simulink model "MyComplexModel_V13R2023a"  (R2023a)
settings: Solver=ode23tb  StartTime=0.0  StopTime=30  FixedStep=0.001  MaxStep=0.001  RelTol=1e-6
values from neighbouring files (symbols this model uses):
  alpha_IS = 30 / (V30_IS.^beta_IS)    [run_one_case_conditional_sampling_pediatric_noVAD_linear.m]    (also in run_one_case_pediatric_noVAD_linear.m)
  alpha_LA = 30 / (V30_LA.^beta_LA)    [run_one_case_conditional_sampling_pediatric_noVAD_linear.m]    (also in run_one_case_pediatric_noVAD_linear.m)
  alpha_LV = 30 / (V30_LV.^beta_LV)    [run_one_case_conditional_sampling_pediatric_noVAD_linear.m]    (also in run_one_case_pediatric_noVAD_linear.m)
  alpha_RA = 30 / (V30_RA.^beta_RA)    [run_one_case_conditional_sampling_pediatric_noVAD_linear.m]    (also in run_one_case_pediatric_noVAD_linear.m)
  alpha_RV = 30 / (V30_RV.^beta_RV)    [run_one_case_conditional_sampling_pediatric_noVAD_linear.m]    (also in run_one_case_pediatric_noVAD_linear.m)
  beta_IS = (log(Pm_IS / 30)) / (log(Vm_IS / V30_IS))    [run_one_case_conditional_sampling_pediatric_noVAD_linear.m]    (also in run_one_case_pediatric_noVAD_linear.m)
  beta_LA = (log(Pm_LA / 30)) / (log(Vm_LA / V30_LA))    [run_one_case_conditional_sampling_pediatric_noVAD_linear.m]    (also in run_one_case_pediatric_noVAD_linear.m)
  beta_LV = (log(Pm_LV / 30)) / (log(Vm_LV / V30_LV))    [run_one_case_conditional_sampling_pediatric_noVAD_linear.m]    (also in run_one_case_pediatric_noVAD_linear.m)
  beta_RA = (log(Pm_RA / 30)) / (log(Vm_RA / V30_RA))    [run_one_case_conditional_sampling_pediatric_noVAD_linear.m]    (also in run_one_case_pediatric_noVAD_linear.m)
  beta_RV = (log(Pm_RV / 30)) / (log(Vm_RV / V30_RV))    [run_one_case_conditional_sampling_pediatric_noVAD_linear.m]    (also in run_one_case_pediatric_noVAD_linear.m)
  C_can_H = 5e-6    (= 5e-06)    [run_one_case_conditional_sampling_pediatric_noVAD_linear.m]    (also in run_one_case_pediatric_noVAD_linear.m)
  Cla = 1.6 * 2    (= 3.2)    [run_one_case_conditional_sampling_pediatric_noVAD_linear.m]    (also in run_one_case_pediatric_noVAD_linear.m)
  Cpulmart = SV_RV / (sPAP - dPAP) * 0.65    [run_one_case_conditional_sampling_pediatric_noVAD_linear.m]    (also in run_one_case_pediatric_noVAD_linear.m = 0.830555555556)
  Cpulmven = Cpulm - Cpulmart    [run_one_case_conditional_sampling_pediatric_noVAD_linear.m]    (also in run_one_case_pediatric_noVAD_linear.m)
  Cra = 4.2 * 2    (= 8.4)    [run_one_case_conditional_sampling_pediatric_noVAD_linear.m]    (also in run_one_case_pediatric_noVAD_linear.m)
  Csysart = SV_LV / (SAP - DAP)    [run_one_case_conditional_sampling_pediatric_noVAD_linear.m]    (also in run_one_case_pediatric_noVAD_linear.m = 0.589743589744)
  Csysven = Csys - Csysart    [run_one_case_conditional_sampling_pediatric_noVAD_linear.m]    (also in run_one_case_pediatric_noVAD_linear.m)
  DE = 2 * 0    (= 0)    [run_one_case_conditional_sampling_pediatric_noVAD_linear.m]    (also in run_one_case_pediatric_noVAD_linear.m)
  DR = 3 * 0    (= 0)    [run_one_case_conditional_sampling_pediatric_noVAD_linear.m]    (also in run_one_case_pediatric_noVAD_linear.m)
  DTs = 3 * 0    (= 0)    [run_one_case_conditional_sampling_pediatric_noVAD_linear.m]    (also in run_one_case_pediatric_noVAD_linear.m)
  DTv = 0.5 * 0    (= 0)    [run_one_case_conditional_sampling_pediatric_noVAD_linear.m]    (also in run_one_case_pediatric_noVAD_linear.m)
  DV = 5 * 0    (= 0)    [run_one_case_conditional_sampling_pediatric_noVAD_linear.m]    (also in run_one_case_pediatric_noVAD_linear.m)
  Emax_LV = 0.5    [run_one_case_conditional_sampling_pediatric_noVAD_linear.m]    (also in run_one_case_pediatric_noVAD_linear.m)
  Emax_RV = 0.5    [run_one_case_conditional_sampling_pediatric_noVAD_linear.m]    (also in run_one_case_pediatric_noVAD_linear.m)
  Emin_LV = -0.5    [run_one_case_conditional_sampling_pediatric_noVAD_linear.m]    (also in run_one_case_pediatric_noVAD_linear.m)
  Emin_RV = -0.5    [run_one_case_conditional_sampling_pediatric_noVAD_linear.m]    (also in run_one_case_pediatric_noVAD_linear.m)
  ESP_LA = LAP * 1.2    [run_one_case_conditional_sampling_pediatric_noVAD_linear.m]    (also in run_one_case_pediatric_noVAD_linear.m = 22.8)
  ESP_LV = k_ESP_LV * SAP    [run_one_case_conditional_sampling_pediatric_noVAD_linear.m]    (also in run_one_case_pediatric_noVAD_linear.m)
  ESP_RA = CVP * 1.2    [run_one_case_conditional_sampling_pediatric_noVAD_linear.m]    (also in run_one_case_pediatric_noVAD_linear.m = 12)
  ESP_RV = k_ESP_RV * sPAP    [run_one_case_conditional_sampling_pediatric_noVAD_linear.m]    (also in run_one_case_pediatric_noVAD_linear.m)
  ESV_LA = EDV_LA - SV_LA    [run_one_case_conditional_sampling_pediatric_noVAD_linear.m]    (also in run_one_case_pediatric_noVAD_linear.m = 59.75)
  ESV_LV = get_required_scalar(sample_row, {'ESVLV', 'ESV_LV'})    [run_one_case_conditional_sampling_pediatric_noVAD_linear.m]    (also in run_one_case_pediatric_noVAD_linear.m = 76)
  ESV_RA = EDV_RA - SV_RA    [run_one_case_conditional_sampling_pediatric_noVAD_linear.m]    (also in run_one_case_pediatric_noVAD_linear.m = 30.05)
  ESV_RV = get_required_scalar(sample_row, {'ESVRV', 'ESV_RV'})    [run_one_case_conditional_sampling_pediatric_noVAD_linear.m]    (also in run_one_case_pediatric_noVAD_linear.m = 40)
  GaE = 0.012    [run_one_case_conditional_sampling_pediatric_noVAD_linear.m]    (also in run_one_case_pediatric_noVAD_linear.m)
  GaR = 0.1    [run_one_case_conditional_sampling_pediatric_noVAD_linear.m]    (also in run_one_case_pediatric_noVAD_linear.m)
  GaTs = 0.015    [run_one_case_conditional_sampling_pediatric_noVAD_linear.m]    (also in run_one_case_pediatric_noVAD_linear.m)
  GaTv = 0.028    [run_one_case_conditional_sampling_pediatric_noVAD_linear.m]    (also in run_one_case_pediatric_noVAD_linear.m)
  GaV = 9.29    [run_one_case_conditional_sampling_pediatric_noVAD_linear.m]    (also in run_one_case_pediatric_noVAD_linear.m)
  GpE = 0    [run_one_case_conditional_sampling_pediatric_noVAD_linear.m]    (also in run_one_case_pediatric_noVAD_linear.m)
  GpR = 0.33    [run_one_case_conditional_sampling_pediatric_noVAD_linear.m]    (also in run_one_case_pediatric_noVAD_linear.m)
  GpTs = 0    [run_one_case_conditional_sampling_pediatric_noVAD_linear.m]    (also in run_one_case_pediatric_noVAD_linear.m)
  GpTv = 0.25    [run_one_case_conditional_sampling_pediatric_noVAD_linear.m]    (also in run_one_case_pediatric_noVAD_linear.m)
  GpV = 0    [run_one_case_conditional_sampling_pediatric_noVAD_linear.m]    (also in run_one_case_pediatric_noVAD_linear.m)
  hr = get_required_scalar(sample_row, {'hr'})    [run_one_case_conditional_sampling_pediatric_noVAD_linear.m]    (also in run_one_case_pediatric_noVAD_linear.m = 112)
  kELV = (Emax_LV - Emin_LV) / (4 * SE0)    (= 0.25)    [run_one_case_conditional_sampling_pediatric_noVAD_linear.m]    (also in run_one_case_pediatric_noVAD_linear.m)
  kERV = (Emax_RV - Emin_RV) / (4 * SE0)    (= 0.25)    [run_one_case_conditional_sampling_pediatric_noVAD_linear.m]    (also in run_one_case_pediatric_noVAD_linear.m)
  kR = (Rmax - Rmin) / (4 * SR0)    (= 0.174809457508)    [run_one_case_conditional_sampling_pediatric_noVAD_linear.m]    (also in run_one_case_pediatric_noVAD_linear.m)
  kT = (Tmax - Tmin) / (4 * ST0)    (= 0.252)    [run_one_case_conditional_sampling_pediatric_noVAD_linear.m]    (also in run_one_case_pediatric_noVAD_linear.m)
  kV = (Vmax - Vmin) / (4 * SV0) / 100    (= 1.75)    [run_one_case_conditional_sampling_pediatric_noVAD_linear.m]    (also in run_one_case_pediatric_noVAD_linear.m)
  L = 1e-6    (= 1e-06)    [Simulink_vars_code.m]    (also in run_one_case_conditional_sampling_pediatric_noVAD_linear.m; run_one_case_pediatric_noVAD_linear.m)
  Lav = Lav / fct    (= 5.64234254909e-06)    [run_one_case_conditional_sampling_pediatric_noVAD_linear.m]    (also in run_one_case_pediatric_noVAD_linear.m)
  Lmv = Lmv / fct    (= 3.13989149577e-06)    [run_one_case_conditional_sampling_pediatric_noVAD_linear.m]    (also in run_one_case_pediatric_noVAD_linear.m)
  Lpv = Lpv / fct    (= 5.14307516405e-06)    [run_one_case_conditional_sampling_pediatric_noVAD_linear.m]    (also in run_one_case_pediatric_noVAD_linear.m)
  Ltv = Ltv / fct    (= 2.29209519806e-06)    [run_one_case_conditional_sampling_pediatric_noVAD_linear.m]    (also in run_one_case_pediatric_noVAD_linear.m)
  mcfp = CO / 60 * Rsysven + CVP    [run_one_case_conditional_sampling_pediatric_noVAD_linear.m]    (also in run_one_case_pediatric_noVAD_linear.m)
  Poffset_IS = Poffset_LV    (= 0)    [run_one_case_conditional_sampling_pediatric_noVAD_linear.m]    (also in run_one_case_pediatric_noVAD_linear.m)
  Poffset_LA = 0    [run_one_case_conditional_sampling_pediatric_noVAD_linear.m]    (also in run_one_case_pediatric_noVAD_linear.m)
  Poffset_LV = 0    [run_one_case_conditional_sampling_pediatric_noVAD_linear.m]    (also in run_one_case_pediatric_noVAD_linear.m)
  Poffset_RA = 0    [run_one_case_conditional_sampling_pediatric_noVAD_linear.m]    (also in run_one_case_pediatric_noVAD_linear.m)
  Poffset_RV = 0    [run_one_case_conditional_sampling_pediatric_noVAD_linear.m]    (also in run_one_case_pediatric_noVAD_linear.m)
  Ps_IS = Ps_LV    [run_one_case_conditional_sampling_pediatric_noVAD_linear.m]    (also in run_one_case_pediatric_noVAD_linear.m)
  Ps_LA = ESP_LA    [run_one_case_conditional_sampling_pediatric_noVAD_linear.m]    (also in run_one_case_pediatric_noVAD_linear.m = 22.8)
  Ps_LV = ESP_LV    [run_one_case_conditional_sampling_pediatric_noVAD_linear.m]    (also in run_one_case_pediatric_noVAD_linear.m)
  Ps_RA = ESP_RA    [run_one_case_conditional_sampling_pediatric_noVAD_linear.m]    (also in run_one_case_pediatric_noVAD_linear.m = 12)
  Ps_RV = ESP_RV    [run_one_case_conditional_sampling_pediatric_noVAD_linear.m]    (also in run_one_case_pediatric_noVAD_linear.m)
  R = 1e-6    (= 1e-06)    [Simulink_vars_code.m]    (also in run_one_case_conditional_sampling_pediatric_noVAD_linear.m; run_one_case_pediatric_noVAD_linear.m)
  Rdir_AV = 0.00375    [run_one_case_conditional_sampling_pediatric_noVAD_linear.m]    (also in run_one_case_pediatric_noVAD_linear.m)
  Rdir_MV = 0.0075    [run_one_case_conditional_sampling_pediatric_noVAD_linear.m]    (also in run_one_case_pediatric_noVAD_linear.m)
  Rdir_PV = 0.00375    [run_one_case_conditional_sampling_pediatric_noVAD_linear.m]    (also in run_one_case_pediatric_noVAD_linear.m)
  Rdir_TV = 0.00375    [run_one_case_conditional_sampling_pediatric_noVAD_linear.m]    (also in run_one_case_pediatric_noVAD_linear.m)
  Rinv_AV = 50    [run_one_case_conditional_sampling_pediatric_noVAD_linear.m]    (also in run_one_case_pediatric_noVAD_linear.m)
  Rinv_MV = 50    [run_one_case_conditional_sampling_pediatric_noVAD_linear.m]    (also in run_one_case_pediatric_noVAD_linear.m)
  Rinv_PV = 50    [run_one_case_conditional_sampling_pediatric_noVAD_linear.m]    (also in run_one_case_pediatric_noVAD_linear.m)
  Rinv_TV = 50    [run_one_case_conditional_sampling_pediatric_noVAD_linear.m]    (also in run_one_case_pediatric_noVAD_linear.m)
  Rmax = (Rsp_max * Rep_max) / (Rsp_max + Rep_max)    (= 1.3359375)    [run_one_case_conditional_sampling_pediatric_noVAD_linear.m]    (also in run_one_case_pediatric_noVAD_linear.m)
  Rmin = (Rsp_min * Rep_min) / (Rsp_min + Rep_min)    (= 0.636699669967)    [run_one_case_conditional_sampling_pediatric_noVAD_linear.m]    (also in run_one_case_pediatric_noVAD_linear.m)
  rpm = 5500    [run_one_case_conditional_sampling_pediatric_noVAD_linear.m]    (also in run_one_case_pediatric_noVAD_linear.m)
  Rpulmart = k_Rpulmart * Rtotpulm    [run_one_case_conditional_sampling_pediatric_noVAD_linear.m]    (also in run_one_case_pediatric_noVAD_linear.m)
  Rpulmven = Rtotpulm - Rpulmart    [run_one_case_conditional_sampling_pediatric_noVAD_linear.m]    (also in run_one_case_pediatric_noVAD_linear.m)
  Rsysart = Rtotsys - Rsysven    [run_one_case_conditional_sampling_pediatric_noVAD_linear.m]    (also in run_one_case_pediatric_noVAD_linear.m)
  Rsysven = k_Rsysven * CO0 / CO    [run_one_case_conditional_sampling_pediatric_noVAD_linear.m]    (also in run_one_case_pediatric_noVAD_linear.m)
  st_a = 0    [conditional_sampling_generate_patients.m]    (also in run_one_case_conditional_sampling_pediatric_noVAD_linear.m; run_one_case_pediatric_noVAD_linear.m)
  st_v = 0    [conditional_sampling_generate_patients.m]    (also in run_one_case_conditional_sampling_pediatric_noVAD_linear.m; run_one_case_pediatric_noVAD_linear.m)
  st_VAD = 0    [conditional_sampling_generate_patients.m]    (also in run_one_case_conditional_sampling_pediatric_noVAD_linear.m; run_one_case_pediatric_noVAD_linear.m)
  st_VADtype = 0    [run_one_case_conditional_sampling_pediatric_noVAD_linear.m]    (also in run_one_case_pediatric_noVAD_linear.m)
  TauE = 1.5    [run_one_case_conditional_sampling_pediatric_noVAD_linear.m]    (also in run_one_case_pediatric_noVAD_linear.m)
  TauR = 1.5    [run_one_case_conditional_sampling_pediatric_noVAD_linear.m]    (also in run_one_case_pediatric_noVAD_linear.m)
  TauTs = 1.8    [run_one_case_conditional_sampling_pediatric_noVAD_linear.m]    (also in run_one_case_pediatric_noVAD_linear.m)
  TauTv = 0.8    [run_one_case_conditional_sampling_pediatric_noVAD_linear.m]    (also in run_one_case_pediatric_noVAD_linear.m)
  TauV = 10    [run_one_case_conditional_sampling_pediatric_noVAD_linear.m]    (also in run_one_case_pediatric_noVAD_linear.m)
  Te = Tresp - Ti    (= 3)    [run_one_case_conditional_sampling_pediatric_noVAD_linear.m]    (also in run_one_case_pediatric_noVAD_linear.m)
  Ti = 2    [run_one_case_conditional_sampling_pediatric_noVAD_linear.m]    (also in run_one_case_pediatric_noVAD_linear.m)
  Tmax = 1.308    [run_one_case_conditional_sampling_pediatric_noVAD_linear.m]    (also in run_one_case_pediatric_noVAD_linear.m)
  Tmin = 0.3    [run_one_case_conditional_sampling_pediatric_noVAD_linear.m]    (also in run_one_case_pediatric_noVAD_linear.m)
  Tresp = 5    [run_one_case_conditional_sampling_pediatric_noVAD_linear.m]    (also in run_one_case_pediatric_noVAD_linear.m)
  V0_LA = 0    [run_one_case_conditional_sampling_pediatric_noVAD_linear.m]    (also in run_one_case_pediatric_noVAD_linear.m)
  V0_LV = 0    [run_one_case_conditional_sampling_pediatric_noVAD_linear.m]    (also in run_one_case_pediatric_noVAD_linear.m)
  V0_RA = 0    [run_one_case_conditional_sampling_pediatric_noVAD_linear.m]    (also in run_one_case_pediatric_noVAD_linear.m)
  V0_RV = 0    [run_one_case_conditional_sampling_pediatric_noVAD_linear.m]    (also in run_one_case_pediatric_noVAD_linear.m)
  Vd_IS = Vd_LV * 0.1    (= 0)    [run_one_case_conditional_sampling_pediatric_noVAD_linear.m]    (also in run_one_case_pediatric_noVAD_linear.m)
  Vd_LA = 0    [run_one_case_conditional_sampling_pediatric_noVAD_linear.m]    (also in run_one_case_pediatric_noVAD_linear.m)
  Vd_LV = 0    [run_one_case_conditional_sampling_pediatric_noVAD_linear.m]    (also in run_one_case_pediatric_noVAD_linear.m)
  Vd_RA = 0    [run_one_case_conditional_sampling_pediatric_noVAD_linear.m]    (also in run_one_case_pediatric_noVAD_linear.m)
  Vd_RV = 0    [run_one_case_conditional_sampling_pediatric_noVAD_linear.m]    (also in run_one_case_pediatric_noVAD_linear.m)
  Vmax = Vusv_max + Vuev_max    (= 2846)    [run_one_case_conditional_sampling_pediatric_noVAD_linear.m]    (also in run_one_case_pediatric_noVAD_linear.m)
  Vmin = Vusv_min + Vuev_min    (= 2146)    [run_one_case_conditional_sampling_pediatric_noVAD_linear.m]    (also in run_one_case_pediatric_noVAD_linear.m)
  Vs_IS = Vs_LV * 0.1    [run_one_case_conditional_sampling_pediatric_noVAD_linear.m]    (also in run_one_case_pediatric_noVAD_linear.m = 11.4)
  Vs_LA = EDV_LA + 5    [run_one_case_conditional_sampling_pediatric_noVAD_linear.m]    (also in run_one_case_pediatric_noVAD_linear.m = 69.35)
  Vs_LV = EDV_LV + 15    [run_one_case_conditional_sampling_pediatric_noVAD_linear.m]    (also in run_one_case_pediatric_noVAD_linear.m = 114)
  Vs_RA = EDV_RA + 5    [run_one_case_conditional_sampling_pediatric_noVAD_linear.m]    (also in run_one_case_pediatric_noVAD_linear.m = 39.65)
  Vs_RV = EDV_RV + 15    [run_one_case_conditional_sampling_pediatric_noVAD_linear.m]    (also in run_one_case_pediatric_noVAD_linear.m = 78)
  Vusv_pulm_ven = k_Vusv_pulm_ven * Vusv_pulm    [run_one_case_conditional_sampling_pediatric_noVAD_linear.m]    (also in run_one_case_pediatric_noVAD_linear.m)
  Vusv_sys_ven = k_Vusv_sys_ven * Vusv_sys    [run_one_case_conditional_sampling_pediatric_noVAD_linear.m]    (also in run_one_case_pediatric_noVAD_linear.m)
undefined symbols (not defined in the file or in its folder): magnitude
libraries: spsMeanLib x9, spsMeanVariableFrequencyLib x5, simulink x3, dspsigops x1
(part 2 of 2)

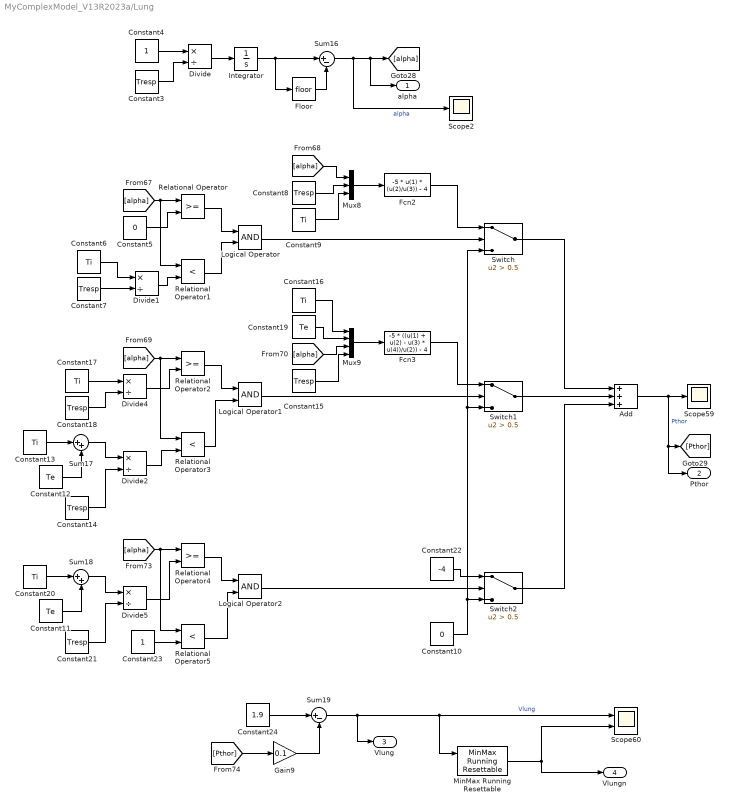
== system MyComplexModel_V13R2023a/Lung ==
  Add : Sum  Inputs=+++
  Constant10 : Constant  Value=0
  Constant11 : Constant  Value=Te
  Constant12 : Constant  Value=Te
  Constant{6,9,13,16..17,20} (6 alike) : Constant  Value=Ti
  Constant{3,7..8,14..15,18,21} (7 alike) : Constant  Value=Tresp
  Constant19 : Constant  Value=Te
  Constant22 : Constant  Value=-4
  Constant23 : Constant
  Constant24 : Constant  Value=1.9
  Constant4 : Constant
  Constant5 : Constant  Value=0
  Divide{,1..2,4..5} (5 alike) : Product  Inputs=*/
  Fcn2 : Fcn  Expr=-5 * u(1) * (u(2)/u(3)) - 4
  Fcn3 : Fcn  Expr=-5 * ((u(1) + u(2) - u(3) * u(4))/u(2)) - 4
  Floor : Rounding
  Gain9 : Gain  Gain=0.1
  Integrator : Integrator
  Logical Operator : Logic  AllPortsSameDT=off  OutDataTypeStr=boolean
  Logical Operator1 : Logic  AllPortsSameDT=off  OutDataTypeStr=boolean
  Logical Operator2 : Logic  AllPortsSameDT=off  OutDataTypeStr=boolean
  MinMax Running Resettable : simulink/Math Operations/MinMax Running Resettable  Function=min  vinit=2.3
  Mux8 : Mux  Inputs=3
  Mux9 : Mux
  Relational Operator : RelationalOperator  OutDataTypeStr=boolean  RndMeth=Simplest  InputSameDT=off
  Relational Operator1 : RelationalOperator  Operator=<  OutDataTypeStr=boolean  RndMeth=Simplest  InputSameDT=off
  Relational Operator2 : RelationalOperator  OutDataTypeStr=boolean  RndMeth=Simplest  InputSameDT=off
  Relational Operator3 : RelationalOperator  Operator=<  OutDataTypeStr=boolean  RndMeth=Simplest  InputSameDT=off
  Relational Operator4 : RelationalOperator  OutDataTypeStr=boolean  RndMeth=Simplest  InputSameDT=off
  Relational Operator5 : RelationalOperator  Operator=<  OutDataTypeStr=boolean  RndMeth=Simplest  InputSameDT=off
  Scope2 : Scope
  Scope59 : Scope
  Scope60 : Scope  NumInputPorts=2
  Sum16 : Sum  Inputs=|+-
  Sum17 : Sum  Inputs=|++
  Sum18 : Sum  Inputs=|++
  Sum19 : Sum  Inputs=|+-
  Switch : Switch  Criteria=u2 > Threshold  Threshold=0.5  SaturateOnIntegerOverflow=off  InputSameDT=off
  Switch1 : Switch  Criteria=u2 > Threshold  Threshold=0.5  SaturateOnIntegerOverflow=off  InputSameDT=off
  Switch2 : Switch  Criteria=u2 > Threshold  Threshold=0.5  SaturateOnIntegerOverflow=off  InputSameDT=off
  alpha : Outport
  Pthor : Outport  Port=2
  Vlung : Outport  Port=3
  Vlungn : Outport  Port=4
  wires:
  [alpha] -> Mux8/1
  Constant22/1 -> Switch2/1
  [alpha] -> Relational Operator/1, Relational Operator1/1
  Relational Operator5/1 -> Logical Operator2/2
  Relational Operator3/1 -> Logical Operator1/2
  Relational Operator1/1 -> Logical Operator/2
  [alpha] -> Relational Operator2/1, Relational Operator3/1
  Sum19/1 -> Vlung/1, MinMax Running Resettable/1, Scope60/1  "Vlung"
  Divide4/1 -> Relational Operator2/2
  Switch/1 -> Add/1
  Floor/1 -> Sum16/2
  Mux8/1 -> Fcn2/1
  [alpha] -> Relational Operator4/1, Relational Operator5/1
  Logical Operator/1 -> Switch/2
  [Pthor] -> Gain9/1
  Constant6/1 -> Divide1/1
  Constant16/1 -> Mux9/1
  Constant10/1 -> Switch/3, Switch1/3, Switch2/3
  Constant19/1 -> Mux9/2
  Relational Operator4/1 -> Logical Operator2/1
  Divide5/1 -> Relational Operator4/2
  Divide1/1 -> Relational Operator1/2
  Sum16/1 -> Scope2/1, alpha/1, [alpha]  "alpha"
  Constant20/1 -> Sum18/1
  Constant24/1 -> Sum19/1
  Fcn3/1 -> Switch1/1
  [alpha] -> Mux9/3
  Add/1 -> Pthor/1, [Pthor], Scope59/1  "Pthor"
  Gain9/1 -> Sum19/2
  Constant7/1 -> Divide1/2
  Constant18/1 -> Divide4/2
  Integrator/1 -> Floor/1, Sum16/1
  Constant11/1 -> Sum18/2
  Mux9/1 -> Fcn3/1
  Constant8/1 -> Mux8/2
  Constant5/1 -> Relational Operator/2
  Fcn2/1 -> Switch/1
  Sum17/1 -> Divide2/1
  Constant13/1 -> Sum17/1
  Constant3/1 -> Divide/2
  Logical Operator2/1 -> Switch2/2
  Constant21/1 -> Divide5/2
  Sum18/1 -> Divide5/1
  Switch2/1 -> Add/3
  Constant23/1 -> Relational Operator5/2
  Switch1/1 -> Add/2
  Divide/1 -> Integrator/1
  Constant17/1 -> Divide4/1
  Relational Operator2/1 -> Logical Operator1/1
  Constant12/1 -> Sum17/2
  Constant4/1 -> Divide/1
  Divide2/1 -> Relational Operator3/2
  Logical Operator1/1 -> Switch1/2
  Constant14/1 -> Divide2/2
  Relational Operator/1 -> Logical Operator/1
  Constant15/1 -> Mux9/4
  Constant9/1 -> Mux8/3
  MinMax Running Resettable/1 -> Vlungn/1, Scope60/2

== system MyComplexModel_V13R2023a/Mitral Valve ==
  LAP : Inport
  LVP : Inport  Port=2
  Gain : Gain  Gain=1/(Lmv)
  MV Inertiance : Integrator
  Rdir : Gain  Gain=Rdir_MV
  Rinv : Gain  Gain=Rinv_MV
  Sum : Sum  Inputs=+--
  Switch : Switch  Criteria=u2 > Threshold  SaturateOnIntegerOverflow=off  InputSameDT=off
  QLVin : Outport
  wires:
  Rinv/1 -> Switch/3
  Gain/1 -> MV Inertiance/1
  Rdir/1 -> Switch/1
  Sum/1 -> Gain/1
  LVP/1 -> Sum/2
  MV Inertiance/1 -> Rinv/1, Switch/2, Rdir/1, QLVin/1  "QLVin"
  LAP/1 -> Sum/1
  Switch/1 -> Sum/3

== system MyComplexModel_V13R2023a/Pulmonal Valve ==
  RVP : Inport
  PAP : Inport  Port=2
  1/Lpv : Gain  Gain=1/(Lpv)
  Add : Sum  Inputs=+--
  PV Inertiance : Integrator
  Rdir : Gain  Gain=Rdir_PV
  Rinv : Gain  Gain=Rinv_PV
  Switch : Switch  Criteria=u2 > Threshold  SaturateOnIntegerOverflow=off  InputSameDT=off
  Qout : Outport
  wires:
  PAP/1 -> Add/2
  Rinv/1 -> Switch/3
  Rdir/1 -> Switch/1
  Add/1 -> 1/Lpv/1
  RVP/1 -> Add/1
  1/Lpv/1 -> PV Inertiance/1
  Switch/1 -> Add/3
  PV Inertiance/1 -> Qout/1, Switch/2, Rinv/1, Rdir/1  "Qout"

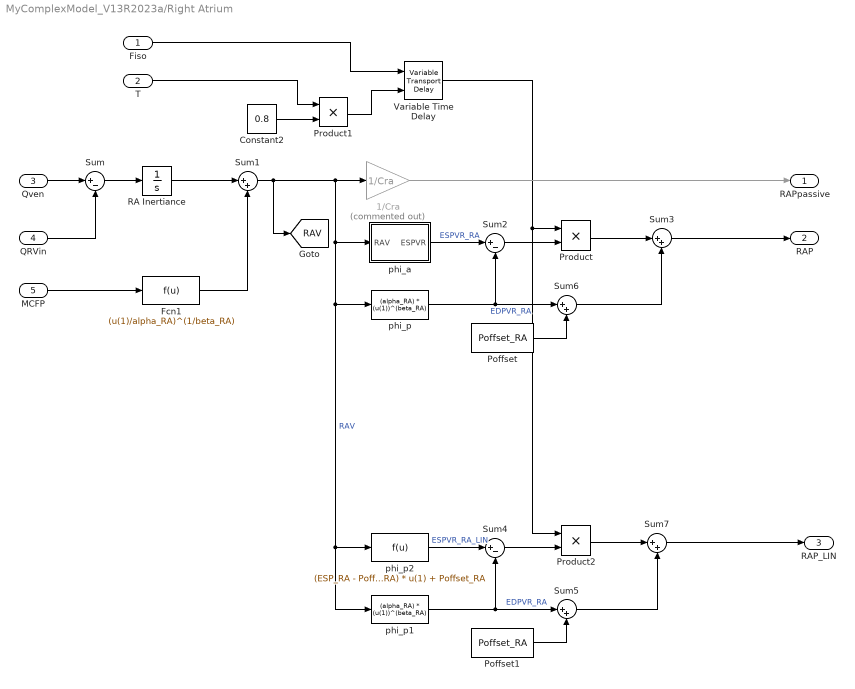
== system MyComplexModel_V13R2023a/Right Atrium ==
  Fiso : Inport
  T : Inport  Port=2
  Qven : Inport  Port=3
  QRVin : Inport  Port=4
  MCFP : Inport  Port=5
  1/Cra : Gain  Commented=on  Gain=1/Cra
  Constant2 : Constant  Value=0.8
  Fcn1 : Fcn  Expr=(u(1)/alpha_RA)^(1/beta_RA)
  Poffset : Constant  Value=Poffset_RA
  Poffset1 : Constant  Value=Poffset_RA
  Product : Product
  Product1 : Product
  Product2 : Product
  RA Inertiance : Integrator
  Sum : Sum  Inputs=|+-
  Sum{1,3,5..7} (5 alike) : Sum  Inputs=|++
  Sum2 : Sum  Inputs=|+-
  Sum4 : Sum  Inputs=|+-
  Variable Time Delay : VariableTransportDelay  MaximumDelay=10
  phi_a : Subsystem
  phi_p : Fcn  Expr=(alpha_RA) * (u(1))^(beta_RA)
  phi_p1 : Fcn  Expr=(alpha_RA) * (u(1))^(beta_RA)
  phi_p2 : Fcn  Expr=(ESP_RA - Poffset_RA)/(ESV_RA - V0_RA) * u(1) + Poffset_RA
  RAPpassive : Outport
  RAP : Outport  Port=2
  RAP_LIN : Outport  Port=3
  tag scope: RAV=global
  wires:
  Constant2/1 -> Product1/2
  Product/1 -> Sum3/1
  phi_a/1(ESPVR) -> Sum2/1  "ESPVR_RA"
  Sum/1 -> RA Inertiance/1
  phi_p/1 -> Sum6/1, Sum2/2  "EDPVR_RA"
  Product1/1 -> Variable Time Delay/2
  Sum2/1 -> Product/2
  T/1 -> Product1/1
  Variable Time Delay/1 -> Product2/1, Product/1
  QRVin/1 -> Sum/2
  Qven/1 -> Sum/1
  Sum3/1 -> RAP/1
  Fiso/1 -> Variable Time Delay/1
  1/Cra/1 -> RAPpassive/1
  RA Inertiance/1 -> Sum1/1
  Fcn1/1 -> Sum1/2
  MCFP/1 -> Fcn1/1
  Sum6/1 -> Sum3/2
  Poffset/1 -> Sum6/2
  Sum1/1 -> [RAV], phi_p2/1, phi_p1/1, phi_p/1, phi_a/1(RAV), 1/Cra/1  "RAV"
  Poffset1/1 -> Sum5/2
  Sum4/1 -> Product2/2
  Product2/1 -> Sum7/1
  Sum5/1 -> Sum7/2
  phi_p2/1 -> Sum4/1  "ESPVR_RA_LIN"
  phi_p1/1 -> Sum5/1, Sum4/2  "EDPVR_RA"
  Sum7/1 -> RAP_LIN/1

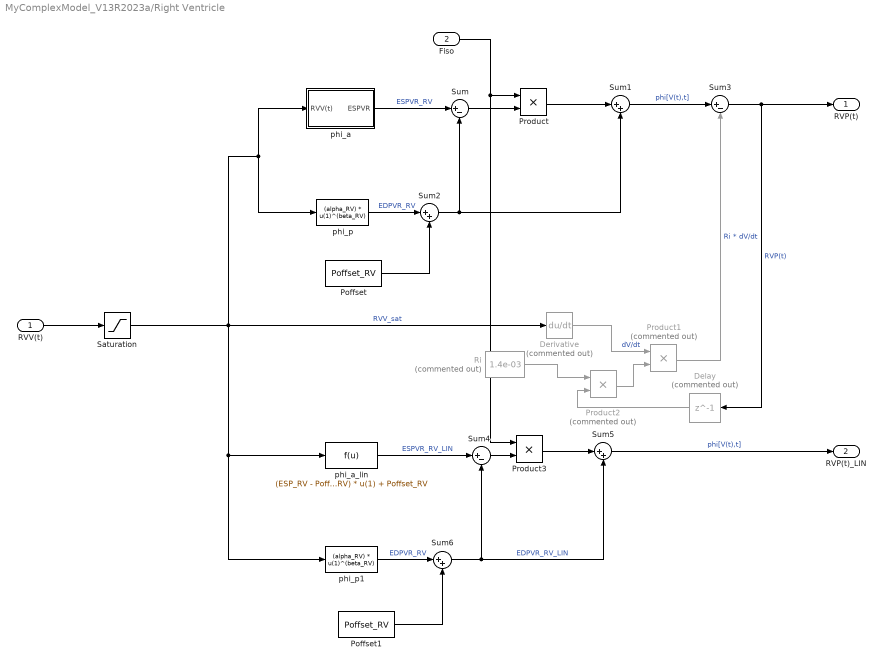
== system MyComplexModel_V13R2023a/Right Ventricle ==
  RVV(t) : Inport
  Fiso : Inport  Port=2
  Delay : Delay  Commented=on  DelayLength=1  InitialCondition=0
  Derivative : Derivative  Commented=on
  Poffset : Constant  Value=Poffset_RV
  Poffset1 : Constant  Value=Poffset_RV
  Product : Product
  Product1 : Product  Commented=on
  Product2 : Product  Commented=on
  Product3 : Product
  Ri : Constant  Commented=on  Value=1.4e-03
  Saturation : Saturate  UpperLimit=Inf  LowerLimit=0
  Sum : Sum  Inputs=|+-
  Sum{1..2,5..6} (4 alike) : Sum  Inputs=|++
  Sum3 : Sum  Inputs=|+-
  Sum4 : Sum  Inputs=|+-
  phi_a : Subsystem
  phi_a_lin : Fcn  Expr=(ESP_RV - Poffset_RV)/(ESV_RV - V0_RV) * u(1) + Poffset_RV
  phi_p : Fcn  Expr=(alpha_RV) * u(1)^(beta_RV)
  phi_p1 : Fcn  Expr=(alpha_RV) * u(1)^(beta_RV)
  RVP(t) : Outport
  RVP(t)_LIN : Outport  Port=2
  wires:
  phi_p/1 -> Sum2/1  "EDPVR_RV"
  phi_a/1(ESPVR) -> Sum/1  "ESPVR_RV"
  Sum/1 -> Product/2
  Fiso/1 -> Product/1, Product3/1
  Product/1 -> Sum1/1
  Sum2/1 -> Sum/2, Sum1/2
  Poffset/1 -> Sum2/2
  Sum1/1 -> Sum3/1  "phi[V(t),t]"
  Sum3/1 -> RVP(t)/1, Delay/1  "RVP(t)"
  Product1/1 -> Sum3/2  "Ri * dV/dt"
  Derivative/1 -> Product1/1  "dV/dt"
  Product2/1 -> Product1/2
  Ri/1 -> Product2/1
  Delay/1 -> Product2/2
  RVV(t)/1 -> Saturation/1
  phi_p1/1 -> Sum6/1  "EDPVR_RV"
  phi_a_lin/1 -> Sum4/1  "ESPVR_RV_LIN"
  Sum4/1 -> Product3/2
  Product3/1 -> Sum5/1
  Poffset1/1 -> Sum6/2
  Sum6/1 -> Sum4/2, Sum5/2  "EDPVR_RV_LIN"
  Sum5/1 -> RVP(t)_LIN/1  "phi[V(t),t]"
  Saturation/1 -> phi_a_lin/1, phi_p1/1, phi_p/1, phi_a/1(RVV(t)), Derivative/1  "RVV_sat"

== system MyComplexModel_V13R2023a/Times ==
  HR : Inport
  Constant : Constant  Value=0.32
  Constant1 : Constant  Value=60
  Constant2 : Constant  Value=-0.01207
  Constant3 : Constant  Value=0.42
  Constant4 : Constant
  Constant5 : Constant  Value=-0.038
  Divide : Product  Inputs=*/
  Divide1 : Product  Inputs=*/
  Fcn : Fcn  Expr=0.5*(exp(u(1)*(u(3)-40))+exp(u(2)*(u(3)-40)))
  Gain : Gain  Gain=2/3
  Mux : Mux  Inputs=3
  Product : Product
  Sum1 : Sum  Inputs=|+-
  Sum2 : Sum  Inputs=|+-
  T : Outport
  Tdia : Outport  Port=2
  Tsys : Outport  Port=3
  Trise : Outport  Port=4
  Tfall : Outport  Port=5
  Xrise : Outport  Port=6
  Yrise : Outport  Port=7
  slope : Outport  Port=8
  wires:
  Sum1/1 -> Sum2/1, Gain/1, Tsys/1  "Tsys"
  Constant1/1 -> Divide/1
  Divide/1 -> Sum1/1, T/1
  HR/1 -> Divide/2, Mux/3
  Constant2/1 -> Mux/1
  Mux/1 -> Fcn/1
  Gain/1 -> Trise/1, Sum2/2, Product/1, Divide1/2
  Sum2/1 -> Tfall/1
  Constant/1 -> Product/2
  Product/1 -> Xrise/1
  Constant3/1 -> Yrise/1
  Constant4/1 -> Divide1/1
  Divide1/1 -> slope/1
  Fcn/1 -> Tdia/1, Sum1/2
  Constant5/1 -> Mux/2

== system MyComplexModel_V13R2023a/Tricuspid Valve ==
  RAP : Inport
  RVP : Inport  Port=2
  1/Ltv : Gain  Gain=1/(Ltv)
  Rdir : Gain  Gain=Rdir_TV
  Rinv : Gain  Gain=Rinv_TV
  Sum : Sum  Inputs=+--
  Switch : Switch  Criteria=u2 > Threshold  SaturateOnIntegerOverflow=off  InputSameDT=off
  TV Inertiance : Integrator
  QRVin : Outport
  wires:
  RAP/1 -> Sum/1
  RVP/1 -> Sum/2
  Rdir/1 -> Switch/1
  Rinv/1 -> Switch/3
  TV Inertiance/1 -> QRVin/1, Rinv/1, Switch/2, Rdir/1  "QLVin"
  1/Ltv/1 -> TV Inertiance/1
  Sum/1 -> 1/Ltv/1
  Switch/1 -> Sum/3

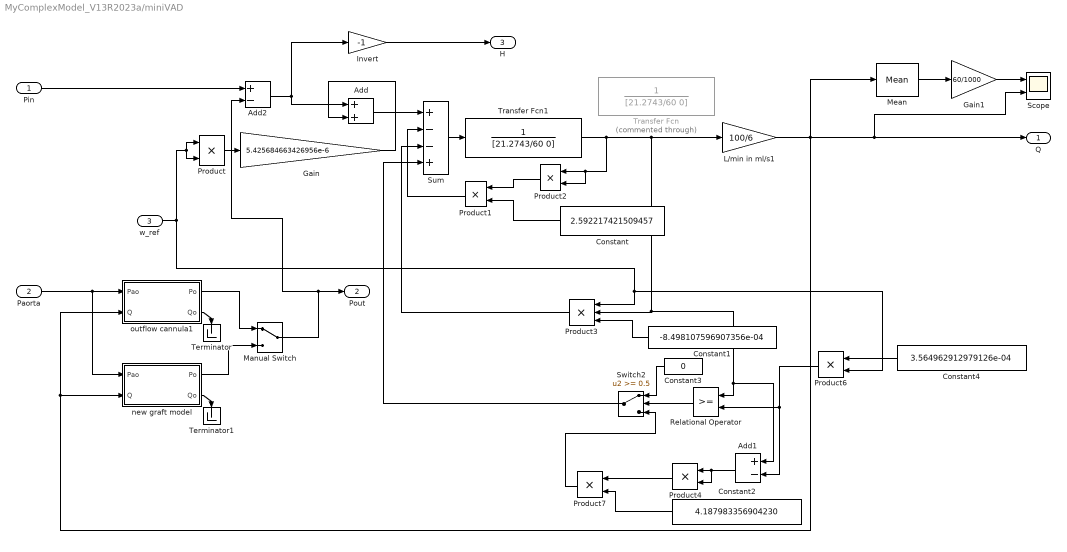
== system MyComplexModel_V13R2023a/miniVAD ==
  Pin : Inport
  Paorta : Inport  Port=2
  w_ref : Inport  Port=3
  Add : Sum
  Add1 : Sum  Inputs=+-
  Add2 : Sum  Inputs=+-
  Constant : Constant  Value=2.592217421509457
  Constant1 : Constant  Value=-8.498107596907356e-04
  Constant2 : Constant  Value=4.187983356904230
  Constant3 : Constant  Value=0
  Constant4 : Constant  Value=3.564962912979126e-04
  Gain : Gain  Gain=5.425684663426956e-6
  Gain1 : Gain  Gain=60/1000
  Invert : Gain  Gain=-1
  L/min in ml/s1 : Gain  Gain=100/6
  Manual Switch : ManualSwitch
  Mean : spsMeanLib/Mean  Freq=hr/60  Vinit=0  Ts=0
  Product{,1..2,4,6..7} (6 alike) : Product  RndMeth=Zero
  Product3 : Product  Inputs=3  RndMeth=Zero
  Relational Operator : RelationalOperator  OutDataTypeStr=boolean  RndMeth=Simplest  InputSameDT=off
  Scope : Scope  NumInputPorts=2
  Sum : Sum  Inputs=+--+
  Switch2 : Switch  Threshold=0.5  ZeroCross=off  SaturateOnIntegerOverflow=off  InputSameDT=off
  Terminator : Terminator
  Terminator1 : Terminator
  Transfer Fcn : TransferFcn  Commented=through  Denominator=[21.2743/60 0]
  Transfer Fcn1 : TransferFcn  Denominator=[21.2743/60 0]
  new graft model : Subsystem
  outflow cannula1 : Subsystem
  Q : Outport  VectorParamsAs1DForOutWhenUnconnected=off
  Pout : Outport  Port=2
  H : Outport  Port=3
  wires:
  Product/1 -> Gain/1
  w_ref/1 -> Product/1, Product/2, Product6/2, Product3/1
  Add/1 -> Sum/1
  Pin/1 -> Add2/1
  Gain/1 -> Add/2
  Sum/1 -> Transfer Fcn1/1
  Product2/1 -> Product1/1
  Product1/1 -> Sum/2
  Product3/1 -> Sum/3
  Constant2/1 -> Product7/2
  Constant1/1 -> Product3/3
  Constant/1 -> Product1/2
  Constant4/1 -> Product6/1
  Relational Operator/1 -> Switch2/2
  Constant3/1 -> Switch2/1
  Product6/1 -> Add1/2, Relational Operator/2
  Add1/1 -> Product4/2, Product4/1
  Product4/1 -> Product7/1
  Product7/1 -> Switch2/3
  Switch2/1 -> Sum/4
  Transfer Fcn1/1 -> Add1/1, Relational Operator/1, Product3/2, L/min in ml/s1/1, Product2/2, Product2/1
  Paorta/1 -> new graft model/1(Pao), outflow cannula1/1(Pao)
  Manual Switch/1 -> Add2/2, Pout/1
  Add2/1 -> Invert/1, Add/1
  Invert/1 -> H/1
  outflow cannula1/2(Qo) -> Terminator/1
  new graft model/2(Qo) -> Terminator1/1
  outflow cannula1/1(Po) -> Manual Switch/1
  new graft model/1(Po) -> Manual Switch/2
  L/min in ml/s1/1 -> Mean/1, Q/1, Scope/2, outflow cannula1/2(Q), new graft model/2(Q)
  Mean/1 -> Gain1/1
  Gain1/1 -> Scope/1

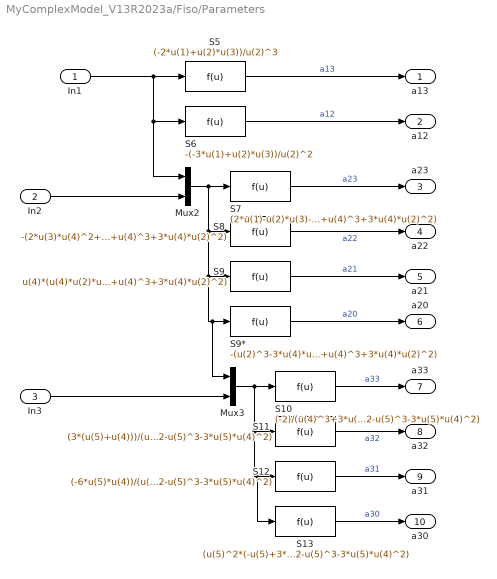
== system MyComplexModel_V13R2023a/Fiso/Parameters ==
  In1 : Inport
  In2 : Inport  Port=2
  In3 : Inport  Port=3
  Mux2 : Mux  Inputs=2
  Mux3 : Mux  Inputs=2
  S10 : Fcn  Expr=(-2)/(u(4)^3+3*u(4)*u(5)^2-u(5)^3-3*u(5)*u(4)^2)
  S11 : Fcn  Expr=(3*(u(5)+u(4)))/(u(4)^3+3*u(4)*u(5)^2-u(5)^3-3*u(5)*u(4)^2)
  S12 : Fcn  Expr=(-6*u(5)*u(4))/(u(4)^3+3*u(4)*u(5)^2-u(5)^3-3*u(5)*u(4)^2)
  S13 : Fcn  Expr=(u(5)^2*(-u(5)+3*u(4)))/(u(4)^3+3*u(4)*u(5)^2-u(5)^3-3*u(5)*u(4)^2)
  S5 : Fcn  Expr=(-2*u(1)+u(2)*u(3))/u(2)^3
  S6 : Fcn  Expr=-(-3*u(1)+u(2)*u(3))/u(2)^2
  S7 : Fcn  Expr=(2*u(1)-u(2)*u(3)-2+u(4)*u(3))/(-u(2)^3-3*u(2)*u(4)^2+u(4)^3+3*u(4)*u(2)^2)
  S8 : Fcn  Expr=-(2*u(3)*u(4)^2+3*u(4)*u(1)-u(4)*u(2)*u(3)-3*u(4)+3*u(2)*u(1)-u(2)^2*u(3)-3*u(2))/(-u(2)^3-3*u(2)*u(4)^2+u(4)^3+3*u(4)*u(2)^2)
  S9 : Fcn  Expr=u(4)*(u(4)*u(2)*u(3)+u(3)*u(4)^2+6*u(2)*u(1)-2*u(2)^2*u(3)-6*u(2))/(-u(2)^3-3*u(2)*u(4)^2+u(4)^3+3*u(4)*u(2)^2)
  S9* : Fcn  Expr=-(u(2)^3-3*u(4)*u(2)^2-u(4)^3*u(1)+u(4)^3*u(2)*u(3)+3*u(4)^2*u(2)*u(1)-u(4)^2*u(2)^2*u(3))/(-u(2)^3-3*u(2)*u(4)^2+u(4)^3+3*u(4)*u(2)^2)
  a13 : Outport
  a12 : Outport  Port=2
  a23 : Outport  Port=3
  a22 : Outport  Port=4
  a21 : Outport  Port=5
  a20 : Outport  Port=6
  a33 : Outport  Port=7
  a32 : Outport  Port=8
  a31 : Outport  Port=9
  a30 : Outport  Port=10
  wires:
  Mux2/1 -> Mux3/1, S9*/1, S9/1, S8/1, S7/1
  In1/1 -> S5/1, S6/1, Mux2/1
  S5/1 -> a13/1  "a13"
  S10/1 -> a33/1  "a33"
  Mux3/1 -> S11/1, S12/1, S13/1, S10/1
  S6/1 -> a12/1  "a12"
  S9*/1 -> a20/1  "a20"
  S7/1 -> a23/1  "a23"
  S13/1 -> a30/1  "a30"
  S9/1 -> a21/1  "a21"
  S11/1 -> a32/1  "a32"
  S12/1 -> a31/1  "a31"
  In3/1 -> Mux3/2
  S8/1 -> a22/1  "a22"
  In2/1 -> Mux2/2

== system MyComplexModel_V13R2023a/HM3/outflow cannula1 ==
  note: Qoc
  Pao : Inport
  Q : Inport  Port=2
  Constant : Constant  Value=1.244e-1
  Constant1 : Constant  Value=-1.244e-1
  Divide : Product  Inputs=**
  Gain : Gain  Gain=1/C_can_H
  Gain1 : Gain  Gain=1/0.223
  Integrator : Integrator  InitialCondition=mcfp*C_can_H
  Integrator1 : Integrator
  L/min in ml/s1 : Gain  Gain=100/6
  Product : Product
  Sum : Sum  Inputs=+-
  Sum1 : Sum  Inputs=+--
  Switch : Switch  Criteria=u2 > Threshold  SaturateOnIntegerOverflow=off  InputSameDT=off
  Po : Outport  VectorParamsAs1DForOutWhenUnconnected=off
  Qo : Outport  Port=2  VectorParamsAs1DForOutWhenUnconnected=off
  wires:
  Switch/1 -> Product/2
  Constant1/1 -> Switch/3
  Constant/1 -> Switch/1
  L/min in ml/s1/1 -> Qo/1, Switch/2, Sum/2
  Product/1 -> Sum1/3
  Divide/1 -> Product/1
  Integrator1/1 -> Gain1/1
  Sum1/1 -> Integrator1/1
  Sum/1 -> Integrator/1
  Gain/1 -> Sum1/1, Po/1
  Q/1 -> Sum/1
  Pao/1 -> Sum1/2
  Integrator/1 -> Gain/1
  Gain1/1 -> L/min in ml/s1/1, Divide/1, Divide/2

== system MyComplexModel_V13R2023a/Interventricular Septum/phi_a^-1 ==
  P_IS : Inport
  Constant : Constant
  Constant1 : Constant  Value=Vs_IS
  Constant2 : Constant  Value=Vd_IS
  Constant3 : Constant  Value=Vs_IS
  Gain : Gain  Gain=1/Ps_IS
  Product : Product
  Sqrt : Sqrt
  Sum : Sum  Inputs=|-+
  Sum1 : Sum  Inputs=|+-
  Sum2 : Sum  Inputs=|-+
  V : Outport
  wires:
  P_IS/1 -> Gain/1
  Gain/1 -> Sum/1
  Constant/1 -> Sum/2
  Sum/1 -> Sqrt/1
  Sqrt/1 -> Product/1
  Constant1/1 -> Sum1/1
  Constant2/1 -> Sum1/2
  Sum1/1 -> Product/2
  Product/1 -> Sum2/1
  Constant3/1 -> Sum2/2
  Sum2/1 -> V/1

== system MyComplexModel_V13R2023a/Left Atrium/phi_a ==
  LAV : Inport
  Constant : Constant
  Divide : Product  Inputs=*/
  Magnitude Squared : Math  Operator=magnitude^2
  P* : Constant  Value=Ps_LA
  Product : Product
  Sum : Sum  Inputs=|+-
  Sum1 : Sum  Inputs=|+-
  Sum2 : Sum  Inputs=|+-
  V* : Constant  Value=Vs_LA
  Vd : Constant  Value=Vd_LA
  ESPVR : Outport
  wires:
  Product/1 -> ESPVR/1  "ESPVR"
  Sum1/1 -> Divide/1
  Divide/1 -> Magnitude Squared/1
  P*/1 -> Product/2
  Sum2/1 -> Divide/2
  Sum/1 -> Product/1
  LAV/1 -> Sum1/2
  Vd/1 -> Sum2/2
  Constant/1 -> Sum/1
  Magnitude Squared/1 -> Sum/2
  V*/1 -> Sum2/1, Sum1/1

== system MyComplexModel_V13R2023a/Left Ventricle/phi_a ==
  note: Vd = 4.3*LVM/100; LVM = 175; (Moscato)
      | V0 = 10; (Colacino)
      | P* = 270; (Moscato)
      | P* = 80 - 360 (Colacino)
  LVV : Inport
  Constant : Constant
  Divide : Product  Inputs=*/
  Magnitude Squared : Math  Operator=magnitude^2
  P* : Constant  Value=Ps_LV
  Product : Product
  Sum : Sum  Inputs=|+-
  Sum1 : Sum  Inputs=|+-
  Sum3 : Sum  Inputs=|+-
  V* : Constant  Value=Vs_LV
  Vd : Constant  Value=Vd_LV
  ESPVR : Outport
  wires:
  Constant/1 -> Sum/1
  LVV/1 -> Sum1/2
  V*/1 -> Sum3/1, Sum1/1
  Vd/1 -> Sum3/2
  Sum/1 -> Product/1
  [Ps_LV] -> Product/2
  Product/1 -> ESPVR/1  "ESPVR"
  Sum1/1 -> Divide/1
  Sum3/1 -> Divide/2
  Divide/1 -> Magnitude Squared/1
  Magnitude Squared/1 -> Sum/2

== system MyComplexModel_V13R2023a/Right Atrium/phi_a ==
  RAV : Inport
  Constant : Constant
  Divide : Product  Inputs=*/
  Magnitude Squared : Math  Operator=magnitude^2
  P* : Constant  Value=Ps_RA
  Product : Product
  Sum : Sum  Inputs=|+-
  Sum1 : Sum  Inputs=|+-
  Sum2 : Sum  Inputs=|+-
  V* : Constant  Value=Vs_RA
  Vd : Constant  Value=Vd_RA
  ESPVR : Outport
  wires:
  Product/1 -> ESPVR/1  "ESPVR"
  Sum1/1 -> Divide/1
  Divide/1 -> Magnitude Squared/1
  P*/1 -> Product/2
  Sum2/1 -> Divide/2
  Sum/1 -> Product/1
  RAV/1 -> Sum1/2
  Vd/1 -> Sum2/2
  Constant/1 -> Sum/1
  Magnitude Squared/1 -> Sum/2
  V*/1 -> Sum2/1, Sum1/1

== system MyComplexModel_V13R2023a/Right Ventricle/phi_a ==
  RVV(t) : Inport
  Constant : Constant
  Divide : Product  Inputs=*/
  Magnitude Squared : Math  Operator=magnitude^2
  P* : Constant  Value=Ps_RV
  Product : Product
  Sum : Sum  Inputs=|+-
  Sum1 : Sum  Inputs=|+-
  Sum2 : Sum  Inputs=|+-
  V* : Constant  Value=Vs_RV
  Vd : Constant  Value=Vd_RV
  ESPVR : Outport
  wires:
  Sum/1 -> Product/1
  Constant/1 -> Sum/1
  V*/1 -> Sum2/1, Sum1/1
  RVV(t)/1 -> Sum1/2
  Sum1/1 -> Divide/1
  Product/1 -> ESPVR/1  "ESPVR"
  Divide/1 -> Magnitude Squared/1
  Vd/1 -> Sum2/2
  Sum2/1 -> Divide/2
  Magnitude Squared/1 -> Sum/2
  [Ps_RV] -> Product/2

== system MyComplexModel_V13R2023a/miniVAD/new graft model ==
  note: Qoc
  Pao : Inport
  Q : Inport  Port=2
  Constant : Constant
  Constant1 : Constant  Value=0
  Divide : Product  Inputs=**
  Gain : Gain  Gain=1/0.001
  Gain1 : Gain  Gain=1/(L/60)
  Gain2 : Gain
  Integrator : Integrator
  Integrator1 : Integrator
  L/min in ml/s1 : Gain  Gain=100/6
  Product : Product
  R : Constant  Value=R
  Sum : Sum  Inputs=+-
  Sum1 : Sum  Inputs=+--
  Switch : Switch  Criteria=u2 > Threshold  SaturateOnIntegerOverflow=off  InputSameDT=off
  Switch1 : Switch  Criteria=u2 > Threshold  SaturateOnIntegerOverflow=off  InputSameDT=off
  Unary Minus : UnaryMinus
  Po : Outport  VectorParamsAs1DForOutWhenUnconnected=off
  Qo : Outport  Port=2  VectorParamsAs1DForOutWhenUnconnected=off
  wires:
  Integrator/1 -> Gain/1
  Gain1/1 -> L/min in ml/s1/1, Divide/2, Divide/1
  Pao/1 -> Sum1/2
  Q/1 -> Sum/1
  Gain/1 -> Sum1/1, Po/1
  Sum/1 -> Integrator/1
  Sum1/1 -> Integrator1/1
  Integrator1/1 -> Gain1/1
  Divide/1 -> Product/1
  Product/1 -> Sum1/3
  L/min in ml/s1/1 -> Sum/2, Switch1/2, Switch/2, Qo/1
  R/1 -> Unary Minus/1, Switch/1
  Unary Minus/1 -> Switch/3
  Switch/1 -> Gain2/1
  Gain2/1 -> Product/2
  Constant/1 -> Switch1/1
  Constant1/1 -> Switch1/3
  Switch1/1 -> ?

== system MyComplexModel_V13R2023a/miniVAD/outflow cannula1 ==
  note: Qoc
  Pao : Inport
  Q : Inport  Port=2
  Constant : Constant  Value=1.244e-1
  Constant1 : Constant  Value=-1.244e-1
  Constant2 : Constant
  Constant3 : Constant  Value=0
  Divide : Product  Inputs=**
  Gain : Gain  Gain=1/0.001
  Gain1 : Gain  Gain=1/(14.15/60)
  Gain2 : Gain
  Integrator : Integrator
  Integrator1 : Integrator
  L/min in ml/s1 : Gain  Gain=100/6
  Product : Product
  Scope : Scope
  Sum : Sum  Inputs=+-
  Sum1 : Sum  Inputs=+--
  Switch : Switch  Criteria=u2 > Threshold  SaturateOnIntegerOverflow=off  InputSameDT=off
  Switch1 : Switch  Criteria=u2 > Threshold  SaturateOnIntegerOverflow=off  InputSameDT=off
  Po : Outport  VectorParamsAs1DForOutWhenUnconnected=off
  Qo : Outport  Port=2  VectorParamsAs1DForOutWhenUnconnected=off
  wires:
  Integrator/1 -> Gain/1
  Gain1/1 -> Scope/1, L/min in ml/s1/1, Divide/1, Divide/2
  Pao/1 -> Sum1/2
  Q/1 -> Sum/1
  Gain/1 -> Sum1/1, Po/1
  Sum/1 -> Integrator/1
  Sum1/1 -> Integrator1/1
  Integrator1/1 -> Gain1/1
  Divide/1 -> Product/1
  Product/1 -> Sum1/3
  Constant/1 -> Switch/1
  Constant1/1 -> Switch/3
  Switch/1 -> Gain2/1
  Gain2/1 -> Product/2
  Constant3/1 -> Switch1/3
  Switch1/1 -> ?
  Constant2/1 -> Switch1/1
  L/min in ml/s1/1 -> Sum/2, Switch/2, Switch1/2, Qo/1
